simulink model "LaneFollowingTestBenchExample"  (R2020a)
settings: Solver=VariableStepAuto  StartTime=0.0  StopTime=simStopTime  RelTol=1e-3
PostLoadFcn:
  | helperLFSetUp
values from neighbouring files (symbols this model uses):
  lr = 1.6    [helperLFSetUp.m]
  m = 1575    [helperLFSetUp.m]
  tau = 0.5    [helperLFSetUp.m]
  Ts = 0.1    [helperLFSetUp.m]
  v_set = egoCar.v0    [helperLFSetUp.m]
undefined symbols (not defined in the file or in its folder): driving
libraries: drivingscenarioandsensors x10, drivinglib x1, autolibshared x1
(part 3 of 3)

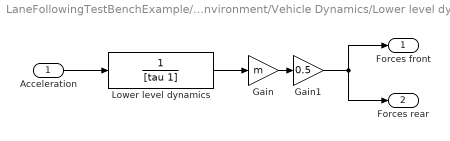
== system LaneFollowingTestBenchExample/Vehicle and Environment/Vehicle Dynamics/Lower level dynamics ==
  Acceleration : Inport
  Gain : Gain  Gain=m
  Gain1 : Gain  Gain=0.5
  Lower level dynamics : TransferFcn  Denominator=[tau 1]
  Forces front : Outport  VectorParamsAs1DForOutWhenUnconnected=off
  Forces rear : Outport  Port=2  VectorParamsAs1DForOutWhenUnconnected=off
  wires:
  Gain/1 -> Gain1/1
  Gain1/1 -> Forces front/1, Forces rear/1
  Acceleration/1 -> Lower level dynamics/1
  Lower level dynamics/1 -> Gain/1

== matlab function LaneFollowingTestBenchExample/Collision Detection/Collision Detection ==
  data: lane input; headway output; actors input; collision output
function [headway,collision] = collisionDetect(lane, actors)

% If lane detection is not available, the ego car is assumed to be located
% in the middle of its lane. The lane width is assumed to be 3.6m, typical
% highway lane width.
laneWidth = 3.6;
halfLaneWidth = laneWidth/2;

% left lane
if lane.Left.Strength > 0.01
    lb = [lane.Left.CurvatureDerivative/6,...
        lane.Left.Curvature/2,...
        lane.Left.HeadingAngle,...
        lane.Left.LateralOffset];
else
    lb = single([0,0,0,halfLaneWidth]);
end

% right lane
if lane.Right.Strength > 0.01
    rb = [lane.Right.CurvatureDerivative/6,...
        lane.Right.Curvature/2,...
        lane.Right.HeadingAngle,...
        lane.Right.LateralOffset];
else
    rb = single([0,0,0,-halfLaneWidth]);    
end

dist = zeros(1,actors.NumActors);

for i = 1:actors.NumActors
    x = actors.Actors(i).Position(1);
    y = actors.Actors(i).Position(2);
    
    yleftLane  = polyval(lb,x);
    yrightLane = polyval(rb,x);
    
    if (yrightLane <= y) && (y <= yleftLane) % within lane boundary?
        dist(i) = hypot(x,y); 
    else
        dist(i) = 100;
    end       
end

headway = min(dist) - 4.7;  % headway from the lead vehicle's trailing surface to the ego vehicle's leading surface
if headway < 1.5
    collision = true; % collision detected
else
    collision = false;
end

== matlab function LaneFollowingTestBenchExample/MIO Track/Pack MIO Track ==
  data: tracks input; mioTrack output Bus: BusMultiObjectTracker1; mioTrackIndex input
function mioTrack = fcn(tracks, mioTrackIndex)
% Extract MIO track and package for visualization in Birds Eye Scope

mioTrack = tracks;

if mioTrackIndex > 0
    % First track represents MIO
    mioTrack.NumTracks = 1;
    mioTrack.Tracks(1) = tracks.Tracks(mioTrackIndex);
else
    % No valid MIO track
    mioTrack.NumTracks = 0;
end

== matlab function LaneFollowingTestBenchExample/Vehicle and Environment/Pack Lanes ==
  data: laneDets input Bus: BusLanes; EgoLane output Bus: BusLaneSensor; NextLane output Bus: BusLaneSensor
%% packLanes
% This function extracts ego and next left lanes and pack them with
%  BusLaneSensor
function [EgoLane,NextLane] = packLanes(laneDets)

numLanes = laneDets.NumLaneBoundaries;
lanes = laneDets.LaneBoundaries;

% read lateral offset for all lanes
offset = zeros(numLanes,1);
for i = 1:numLanes
    offset(i) = lanes(i).LateralOffset;
end

% create dummy lane with zero strength
dummyLane = struct(...
    'Curvature',single(0),...
    'CurvatureDerivative', single(0), ...
    'HeadingAngle', single(0), ...
    'LateralOffset', single(0), ...
    'Strength', single(0));

% sort the lateral offset
rb = sort(offset(offset<=0),'descend');  % right lanes 
lb = sort(offset(offset>0),'ascend');    % left lane

if length(lb)>=2 % both left ego and next lanes exist?
    egoLeftIndx = searchIndx(offset, numLanes, lb(1)); % index for ego left lane
    EgoLane.Left = getLaneParameters(lanes(egoLeftIndx));

    nextLeftIndx = searchIndx(offset, numLanes, lb(2)); % index for left next lane  
    NextLane.Left = getLaneParameters(lanes(nextLeftIndx));
elseif length(lb)==1 % no left next lane, only left ego lane?
    egoLeftIndx = searchIndx(offset, numLanes, lb(1));  % index for left ego lane 
    EgoLane.Left = getLaneParameters(lanes(egoLeftIndx));
    
    NextLane.Left = dummyLane; % no left next lane
else % no left lanes
    EgoLane.Left = dummyLane;  % no left ego lane
    NextLane.Left = dummyLane; % no left next lane  
end

if length(rb)>=2 % both right ego and next lanes exist?
    egoRightIndx = searchIndx(offset, numLanes, rb(1));  % index for right ego lane   
    EgoLane.Right = getLaneParameters(lanes(egoRightIndx));

    nextRightIndx = searchIndx(offset, numLanes, rb(2)); % index for right next lane      
    NextLane.Right = getLaneParameters(lanes(nextRightIndx));
elseif length(rb)==1 % no right next lane, only right ego lane?
    egoRightIndx = searchIndx(offset, numLanes, rb(1));  % index for right ego lane   
    EgoLane.Right = getLaneParameters(lanes(egoRightIndx));
    
    NextLane.Right = dummyLane; % no right next lane
else % no right lanes
    EgoLane.Right = dummyLane;  % no right ego lane
    NextLane.Right = dummyLane; % no right next lane    
end

end
% Search for next index
function indx = searchIndx(offset, num, val)

indx = 0;
for i = 1:num
    if offset(i) == val
        indx = i;
        return;
    end
end

end

% read laneBoundaries and convert units from deg to rad
function laneSensor = getLaneParameters(LaneBoundaries)

laneSensor.Curvature = single(deg2rad(LaneBoundaries.Curvature));
laneSensor.CurvatureDerivative = single(deg2rad(LaneBoundaries.CurvatureDerivative));
laneSensor.HeadingAngle = single(deg2rad(LaneBoundaries.HeadingAngle));
laneSensor.LateralOffset = single(LaneBoundaries.LateralOffset);
laneSensor.Strength = single(LaneBoundaries.Strength);

end

== matlab function LaneFollowingTestBenchExample/Vehicle and Environment/Pack Ego Actor ==
  data: pos input; a output Bus: BusActors1Actors size=1; vel input; yaw input; yawRate input
function a = packEgo(pos,vel,yaw,yawRate)
% Pack ego information into a single ego actor bus
%
% Imoprtant note:
% Output is a bus of type BusActorsActors. This is the same bus used by the
% Scenario Reader to output an individual actor. If you change the
% output bus name of Scenario Reader change the output bus name here
% as well by clicking on 'Edit Data' in the menu above.

a = struct(...
    'ActorID',1,...
    'Position', [pos(1) pos(2) 0], ...
    'Velocity', [vel(1) vel(2) 0], ...
    'Roll', 0, ...
    'Pitch', 0, ...
    'Yaw', yaw, ...
    'AngularVelocity', [0 0 yawRate]);
